simulink model "q_heli3d_skeleton_2012b"
settings: Solver=ode1  StartTime=0.0  StopTime=inf  FixedStep=0.002  RelTol=1e-3
undefined symbols (not defined in the file): A, B, C, C_0, CMD_ELEV_POS_LIMIT_LOWER, CMD_ELEV_POS_LIMIT_UPPER, CMD_RATE_LIMIT, CMD_TRAVEL_POS_LIMIT_LOWER, CMD_TRAVEL_POS_LIMIT_UPPER, elev_0, HIL, K_AMP, K_EC_E, K_EC_P, K_EC_T, K_i, K_JOYSTICK_X, K_JOYSTICK_Y, K_r, K_sf, L, qc_get_step_size, VMAX_AMP, VMAX_DAC, Vo
libraries: quarc_library x5, simulink x2, simulink_extras x2
settings Model: SimulationMode=external  ExtModeTrigDuration=500000  Creator=MLevis  LastModifiedBy=s4358046
settings SolverCC: PositivePriorityOrder=on
settings DataIOCC: LimitDataPoints=on  SaveFormat=Array  SignalLoggingSaveFormat=ModelDataLogs  ReturnWorkspaceOutputs=off
settings OptimizationCC: ExpressionDepthLimit=2147483647  InitFltsAndDblsToZero=on  LifeSpan=inf  SimCompilerOptimization=Off
settings DebuggingCC: SaveWithParameterizedLinksMsg=none  UnderspecifiedInitializationDetection=Classic  MergeDetectMultiDrivingBlocksExec=none  SolverPrmCheckMsg=warning  MultiTaskDSMMsg=warning  MultiTaskCondExecSysMsg=none  FcnCallInpInsideContextMsg=Enable All  StateNameClashWarn=warning  StrictBusMsg=None  SFUnexpectedBacktrackingDiag=warning  SFNoUnconditionalDefaultTransitionDiag=warning
settings HardwareCC: ProdBitPerPointer=32  ProdLargestAtomicFloat=None  ProdIntDivRoundTo=Undefined  ProdEndianess=Unspecified  ProdWordSize=32  ProdHWDeviceType=32-bit Generic
settings ModelReferenceCC: PropagateSignalLabelsOutOfModel=off
settings SFSimCC: SimUseLocalCustomCode=off
settings RTWCC: SystemTargetFile=quarc_win64.tlc  TemplateMakefile=quarc_default_tmf  Description=QUARC Win64 Target  ProcessScript=quarc_win64_make_rtw_hook  RTWUseLocalCustomCode=off  IncludeERTFirstTime=on  RTWCompilerOptimization=Off
settings CodeAppCC: CustomSymbolStrType=$N$R$M
settings STFCustomTargetCC: TargetPreCompLibLocation=C:\PROGRA~3\QUARC\lib\2012a\win64\release  CodeReplacementLibrary=C89/C90 (ANSI)  GeneratePreprocessorConditionals=Disable all  CombineOutputUpdateFcns=on  GRTInterface=off  SystemTargetFile=quarc_win64.tlc
settings GRTTargetCC: TargetPreCompLibLocation=C:\PROGRA~3\QUARC\lib\2012a\win64\release  CodeReplacementLibrary=C89/C90 (ANSI)  ParMdlRefBuildCompliant=off  CompOptLevelCompliant=off  ConcurrentExecutionCompliant=off  GeneratePreprocessorConditionals=Disable all  MatFileLogging=off  CPPClassGenCompliant=off  ExtMode=on  ExtModeMexFile=quarc_comm

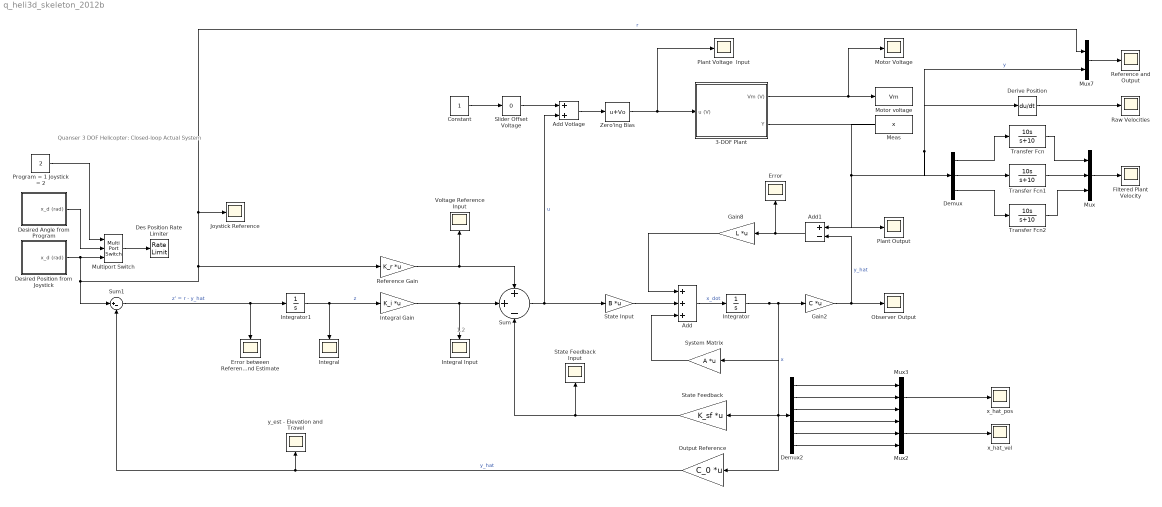
== system q_heli3d_skeleton_2012b ==
  note: Quanser 3 DOF Helicopter:
      | Closed-loop Actual System
  note: 1.2
  3-DOF Plant : Subsystem
  Add : Sum  Inputs=+++
  Add Votlage : Sum
  Add1 : Sum  Inputs=+-
  Constant : Constant
  Demux : Demux  Outputs=3
  Demux2 : Demux  Outputs=6
  Derive Position : Derivative
  Des Position Rate Limiter : RateLimiter  RisingSlewLimit=CMD_RATE_LIMIT  FallingSlewLimit=-CMD_RATE_LIMIT  SampleTimeMode=inherited
  Desired Angle from Program : Subsystem
  Desired Position from Joystick : Subsystem
  Error : Scope
      settings: TimeRange=10  YMin=-0.00225  YMax=0.002  SaveName=Error
  Error between Reference and Estimate : Scope
      settings: TimeRange=10  YMin=-0.01  YMax=0.06  SaveName=int_err
  Filtered Plant Velocity : Scope
      settings: YMin=-1.75  YMax=1.75  SaveName=y_plant_vel_filt
  Gain2 : Gain  Gain=C  Multiplication=Matrix(K*u)
  Gain8 : Gain  Gain=L  Multiplication=Matrix(K*u)
  Integral : Scope
      settings: TimeRange=10  YMin=-0.05  YMax=0.325  SaveName=int_input1
  Integral Gain : Gain  Gain=K_i  Multiplication=Matrix(K*u)
  Integral Input : Scope
      settings: TimeRange=10  YMin=-6  YMax=10  SaveName=int_input
  Integrator : Integrator
  Integrator1 : Integrator  LimitOutput=on  UpperSaturationLimit=0.7  LowerSaturationLimit=-0.7
  Joystick Reference : Scope
      settings: TimeRange=10  YMin=-0.1  YMax=2.2  SaveName=ref_info
  Meas : ToWorkspace  VariableName=x  SampleTime=-1
  Motor Voltage : Scope
      settings: YMin=-0.5  YMax=0.25  SaveName=Motor_Voltage
  Motor voltage : ToWorkspace  VariableName=Vm  SampleTime=-1
  Multiport Switch : MultiPortSwitch  Inputs=2  zeroidx=off
  Mux : Mux  Inputs=3
  Mux2 : Mux  Inputs=3
  Mux3 : Mux  Inputs=3
  Mux7 : Mux  Inputs=2
  Observer Output : Scope
      settings: TimeRange=10  YMin=-0.5  YMax=0.15  SaveName=y_est
  Output Reference : Gain  Gain=C_0  Multiplication=Matrix(K*u)
  Plant Output : Scope
      settings: YMin=-0.25  YMax=2.25  SaveName=y_plant_pos
  Plant Voltage  Input : Scope
      settings: TimeRange=10  YMin=1.3  YMax=2.9  SaveName=plnt_input
  Program = 1 Joystick = 2 : Constant  Value=2
  Raw Velocities : Scope
      settings: YMin=-0.8  YMax=0.8  SaveName=y_plant_vel
  Reference Gain : Gain  Gain=K_r  Multiplication=Matrix(K*u)
  Reference and Output : Scope
      settings: TimeRange=10  YMin=-0.1  YMax=1.2  SaveName=steady_state_error
  Slider Offset Voltage : simulink/Math Operations/Slider Gain  low=0  gain=0  high=4
  State Feedback : Gain  Gain=K_sf  Multiplication=Matrix(K*u)
  State Feedback Input : Scope
      settings: TimeRange=10  YMin=-55  YMax=55  SaveName=sf_input
  State Input : Gain  Gain=B  Multiplication=Matrix(K*u)
  Sum : Sum  Inputs=++-
  Sum1 : Sum  Inputs=|+-
  System Matrix : Gain  Gain=A  Multiplication=Matrix(K*u)
  Transfer Fcn : TransferFcn  Numerator=[10 0]  Denominator=[1 10]
  Transfer Fcn1 : TransferFcn  Numerator=[10 0]  Denominator=[1 10]
  Transfer Fcn2 : TransferFcn  Numerator=[10 0]  Denominator=[1 10]
  Voltage Reference Input : Scope
      settings: TimeRange=10  YMin=-7  YMax=-0.5  SaveName=ref_input
  Zero'ing Bias : Bias  Bias=Vo
  x_hat_pos : Scope
      settings: YMin=-0.05  YMax=0.325  SaveName=x_hat_pos
  x_hat_vel : Scope
      settings: YMin=-1.5  YMax=1.25  SaveName=x_hat_vel
  y_est - Elevation and Travel : Scope
      settings: YMin=-0.7  YMax=0.2  SaveName=y_est_e_t
  wires:
  Program = 1 Joystick = 2/1 -> Multiport Switch/1
  Desired Position from Joystick/1(x_d (rad)) -> Multiport Switch/3, Sum1/1, Mux7/1, Joystick Reference/1, Reference Gain/1  "r"
  Multiport Switch/1 -> Des Position Rate Limiter/1
  3-DOF Plant/1(Vm (V)) -> Motor voltage/1, Motor Voltage/1
  Zero'ing Bias/1 -> Plant Voltage  Input/1, 3-DOF Plant/1(u (V))
  Desired Angle from Program/1(x_d (rad)) -> Multiport Switch/2
  Transfer Fcn/1 -> Mux/1
  Demux/1 -> Transfer Fcn/1
  Demux/2 -> Transfer Fcn1/1
  Transfer Fcn1/1 -> Mux/2
  Demux/3 -> Transfer Fcn2/1
  Transfer Fcn2/1 -> Mux/3
  Mux/1 -> Filtered Plant Velocity/1
  State Input/1 -> Add/2
  Add/1 -> Integrator/1  "x_dot"
  System Matrix/1 -> Add/3
  Integrator/1 -> System Matrix/1, Gain2/1, Output Reference/1, State Feedback/1, Demux2/1  "x"
  Gain2/1 -> Observer Output/1, Add1/2  "y_hat"
  Sum/1 -> Add Votlage/2, State Input/1  "u"
  Reference Gain/1 -> Sum/1, Voltage Reference Input/1
  Add1/1 -> Gain8/1, Error/1
  Gain8/1 -> Add/1
  3-DOF Plant/2(Y) -> Meas/1, Derive Position/1, Demux/1, Mux7/2, Plant Output/1, Add1/1  "y"
  Demux2/4 -> Mux2/1
  Demux2/5 -> Mux2/2
  Demux2/6 -> Mux2/3
  Demux2/1 -> Mux3/1
  Demux2/2 -> Mux3/2
  Demux2/3 -> Mux3/3
  Mux3/1 -> x_hat_pos/1
  Mux2/1 -> x_hat_vel/1
  Derive Position/1 -> Raw Velocities/1
  Output Reference/1 -> Sum1/2, y_est - Elevation and Travel/1  "y_hat"
  Sum1/1 -> Integrator1/1, Error between Reference and Estimate/1  "z' = r - y_hat"
  State Feedback/1 -> State Feedback Input/1, Sum/3
  Integrator1/1 -> Integral/1, Integral Gain/1  "z"
  Constant/1 -> Slider Offset Voltage/1
  Add Votlage/1 -> Zero'ing Bias/1
  Slider Offset Voltage/1 -> Add Votlage/1
  Integral Gain/1 -> Integral Input/1, Sum/2
  Mux7/1 -> Reference and Output/1

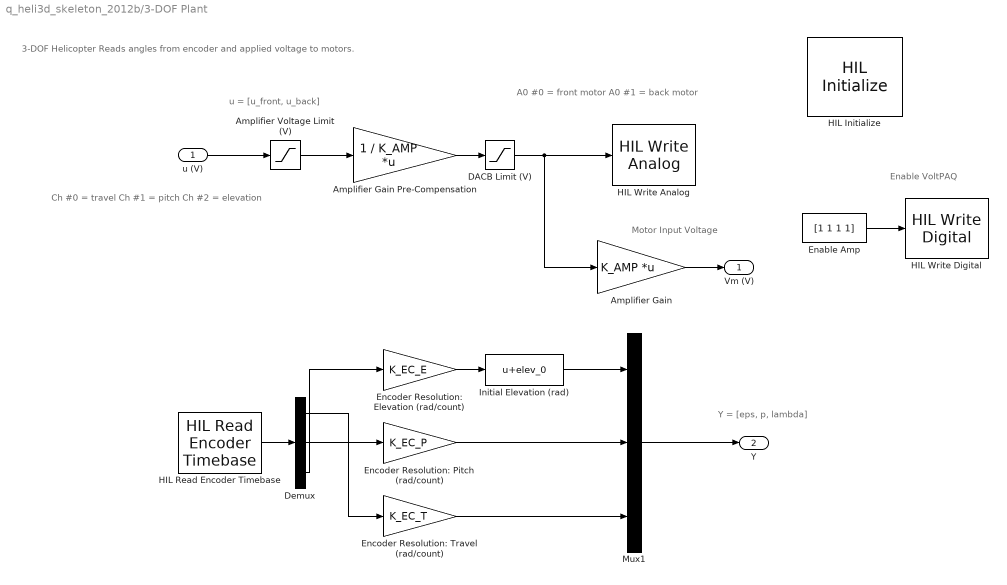
== system q_heli3d_skeleton_2012b/3-DOF Plant ==
  note: A0 #0 = front motor
      | A0 #1 = back motor
  note: u = [u_front, u_back]
  note: Motor Input Voltage
  note: 3-DOF Helicopter
      | Reads angles from encoder and applied voltage to motors.
  note: Ch #0 = travel
      | Ch #1 = pitch
      | Ch #2 = elevation
  note: Y = [eps, p, lambda]
  note: Enable VoltPAQ
  u (V) : Inport
  Amplifier Gain : Gain  Gain=K_AMP  Multiplication=Matrix(K*u)  SaturateOnIntegerOverflow=on  OutDataTypeStr=Inherit: Same as input  ParamDataTypeStr=Inherit: Same as input
  Amplifier Gain Pre-Compensation : Gain  Gain=1 / K_AMP  Multiplication=Matrix(K*u)  SaturateOnIntegerOverflow=on  OutDataTypeStr=Inherit: Same as input  ParamDataTypeStr=Inherit: Same as input
  Amplifier Voltage Limit (V) : Saturate  UpperLimit=VMAX_AMP  LowerLimit=-VMAX_AMP
  DACB Limit (V) : Saturate  UpperLimit=VMAX_DAC  LowerLimit=-VMAX_DAC
  Demux : Demux  Outputs=3
  Enable Amp : Constant  Value=[1 1 1 1]
  Encoder Resolution: Elevation (rad/count) : Gain  Gain=K_EC_E
  Encoder Resolution: Pitch (rad/count) : Gain  Gain=K_EC_P
  Encoder Resolution: Travel (rad/count) : Gain  Gain=K_EC_T
  HIL Initialize : quarc_library/Data Acquisition/Generic/Configuration/HIL Initialize  object_name=HIL-1  board_type=q8_usb  board_number=0  board_options=update_rate=normal  exclusive=off  active=on  hardware_clocks=[0:2]  clock_modes=[]  initial_clock_frequencies=[]  set_clock_params_at_start=off  set_clock_params_at_switch_in=off  set_clock_frequencies_at_start=off  set_clock_frequencies_at_switch_in=off  analog_input_channels=[0:7]  analog_input_maximums=10  analog_input_minimums=-10  set_analog_input_params_at_start=on  set_analog_input_params_at_switch_in=off  analog_output_channels=[0:7]  analog_output_maximums=10  analog_output_minimums=-10  initial_analog_outputs=[0]  final_analog_outputs=[0]  watchdog_analog_outputs=0  set_analog_output_params_at_start=on  set_analog_output_params_at_switch_in=off  set_analog_outputs_at_start=on  set_analog_outputs_at_switch_in=off  set_analog_outputs_at_terminate=on  set_analog_outputs_at_switch_out=off  set_analog_outputs_on_watchdog=off  digital_input_channels=[4:7]  digital_output_channels=[0:3]  digital_output_configuration=[]  initial_digital_outputs=[0]  final_digital_outputs=[0]  watchdog_digital_outputs=[0]  set_digital_output_params_at_start=off  set_digital_output_params_at_switch_in=off  set_digital_outputs_at_start=on  set_digital_outputs_at_switch_in=off  set_digital_outputs_at_terminate=on  set_digital_outputs_at_switch_out=off  set_digital_outputs_on_watchdog=off  encoder_channels=[0:7]  quadrature=[4]  encoder_filter_frequency=[]  initial_encoder_counts=[0]  set_encoder_params_at_start=on  set_encoder_params_at_switch_in=off  set_encoder_counts_at_start=on  set_encoder_counts_at_switch_in=off  pwm_channels=[0:7]  pwm_modes=0  pwm_frequency=99.532799999999995e6/4095  pwm_configuration=[0]  pwm_alignment=[0]  pwm_polarity=[1]  pwm_leading_deadband=[0]  pwm_trailing_deadband=[0]  initial_pwm_outputs=[0]  final_pwm_outputs=[0]  watchdog_pwm_outputs=[0]  set_pwm_params_at_start=on  set_pwm_params_at_switch_in=off  set_pwm_outputs_at_start=on  set_pwm_outputs_at_switch_in=off  set_pwm_outputs_at_terminate=on  set_pwm_outputs_at_switch_out=off  set_pwm_outputs_on_watchdog=off  other_output_channels=[]  initial_other_outputs=[]  final_other_outputs=[]  watchdog_other_outputs=[]  set_other_outputs_at_start=off  set_other_outputs_at_switch_in=off  set_other_outputs_at_terminate=off  set_other_outputs_at_switch_out=off  set_other_outputs_on_watchdog=off
  HIL Read Encoder Timebase : quarc_library/Data Acquisition/Generic/Timebases/HIL Read Encoder Timebase  object_name=HIL-1  clock=0  channels=[0,1,2]  samples_in_buffer=max(ceil(1/qc_get_step_size), 1)  active=on  vector_output=on  data_type_mode=Inherit via back propagation  data_type=double
  HIL Write Analog : quarc_library/Data Acquisition/Generic/Immediate I//O/HIL Write Analog  object_name=HIL-1  channels=[0,1]  sample_time=-1  active=off  vector_input=on
  HIL Write Digital : quarc_library/Data Acquisition/Generic/Immediate I//O/HIL Write Digital  object_name=HIL-1  channels=[0:3]  sample_time=-1  active=off  vector_input=on
  Initial Elevation (rad) : Bias  Bias=elev_0
  Mux1 : Mux  Inputs=3
  Vm (V) : Outport
  Y : Outport  Port=2
  wires:
  HIL Read Encoder Timebase/1 -> Demux/1
  Mux1/1 -> Y/1
  Amplifier Gain Pre-Compensation/1 -> DACB Limit (V)/1
  Amplifier Voltage Limit (V)/1 -> Amplifier Gain Pre-Compensation/1
  Amplifier Gain/1 -> Vm (V)/1
  u (V)/1 -> Amplifier Voltage Limit (V)/1
  DACB Limit (V)/1 -> Amplifier Gain/1, HIL Write Analog/1
  Demux/3 -> Encoder Resolution: Elevation (rad/count)/1
  Demux/1 -> Encoder Resolution: Travel (rad/count)/1
  Demux/2 -> Encoder Resolution: Pitch (rad/count)/1
  Encoder Resolution: Elevation (rad/count)/1 -> Initial Elevation (rad)/1
  Encoder Resolution: Pitch (rad/count)/1 -> Mux1/2
  Encoder Resolution: Travel (rad/count)/1 -> Mux1/3
  Initial Elevation (rad)/1 -> Mux1/1
  Enable Amp/1 -> HIL Write Digital/1

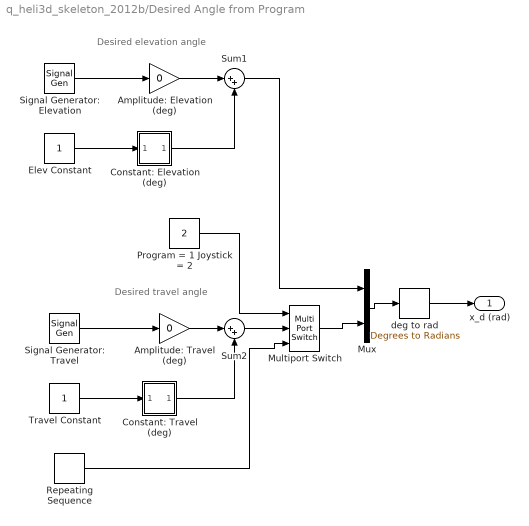
== system q_heli3d_skeleton_2012b/Desired Angle from Program ==
  note: Desired travel angle
  note: Desired elevation angle
  Amplitude: Elevation (deg) : Gain  Gain=0
  Amplitude: Travel (deg) : Gain  Gain=0
  Constant: Elevation (deg) : Subsystem  LoadFcn=slideg Load  StartFcn=slideg StartFcn  StopFcn=slideg StopFcn  mask(Slider Gain){low=-27.5, gain=-27.5, high=30}
      settings: CopyFcn=slideg Copy  DeleteFcn=slideg DeleteBlock  NameChangeFcn=slideg NameChange  OpenFcn=slideg Open  CloseFcn=slideg Close  ParentCloseFcn=slideg ParentClose
      mask Display: disp(gain)
  Constant: Travel (deg) : Subsystem  LoadFcn=slideg Load  StartFcn=slideg StartFcn  StopFcn=slideg StopFcn  mask(Slider Gain){low=-90, gain=0, high=90}
      settings: CopyFcn=slideg Copy  DeleteFcn=slideg DeleteBlock  NameChangeFcn=slideg NameChange  OpenFcn=slideg Open  CloseFcn=slideg Close  ParentCloseFcn=slideg ParentClose
      mask Display: disp(gain)
  Elev Constant : Constant
  Multiport Switch : MultiPortSwitch  Inputs=2  zeroidx=off
  Mux : Mux  Inputs=2
  Program = 1 Joystick = 2 : Constant  Value=2
  Repeating Sequence : simulink/Sources/Repeating Sequence  rep_seq_t="[0  15 16  30  45  46 60 ]"  rep_seq_y="[0 0 30 30  30 0 0 ]"
  Signal Generator: Elevation : SignalGenerator  WaveForm=square  Frequency=0.04
  Signal Generator: Travel : SignalGenerator  WaveForm=square  Frequency=0.03
  Sum1 : Sum  Inputs=|++
  Sum2 : Sum  Inputs=|++
  Travel Constant : Constant
  deg to rad : simulink_extras/Transformations/Degrees to Radians
  x_d (rad) : Outport
  wires:
  deg to rad/1 -> x_d (rad)/1
  Signal Generator: Travel/1 -> Amplitude: Travel (deg)/1
  Amplitude: Travel (deg)/1 -> Sum2/1
  Travel Constant/1 -> Constant: Travel (deg)/1(In1)
  Sum1/1 -> Mux/1
  Signal Generator: Elevation/1 -> Amplitude: Elevation (deg)/1
  Amplitude: Elevation (deg)/1 -> Sum1/1
  Mux/1 -> deg to rad/1
  Elev Constant/1 -> Constant: Elevation (deg)/1(In1)
  Constant: Elevation (deg)/1(Out1) -> Sum1/2
  Constant: Travel (deg)/1(Out1) -> Sum2/2
  Sum2/1 -> Multiport Switch/2
  Repeating Sequence/1 -> Multiport Switch/3
  Multiport Switch/1 -> Mux/2
  Program = 1 Joystick = 2/1 -> Multiport Switch/1

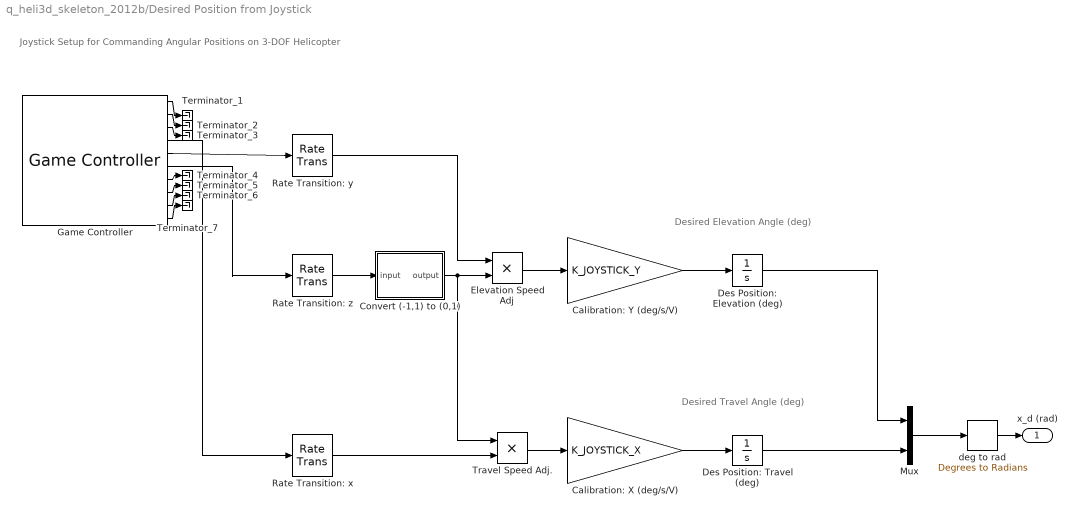
== system q_heli3d_skeleton_2012b/Desired Position from Joystick ==
  note: Desired Elevation Angle (deg)
  note: Desired Travel Angle (deg)
  note: Joystick Setup for Commanding Angular Positions on 3-DOF Helicopter
  Calibration: X (deg/s/V) : Gain  Gain=K_JOYSTICK_X
  Calibration: Y (deg/s/V) : Gain  Gain=K_JOYSTICK_Y
  Convert (-1,1) to (0,1) : Subsystem
  Des Position: Elevation (deg) : Integrator  InitialCondition=elev_0*180/pi  LimitOutput=on  UpperSaturationLimit=CMD_ELEV_POS_LIMIT_UPPER  LowerSaturationLimit=CMD_ELEV_POS_LIMIT_LOWER
  Des Position: Travel (deg) : Integrator  UpperSaturationLimit=CMD_TRAVEL_POS_LIMIT_UPPER  LowerSaturationLimit=CMD_TRAVEL_POS_LIMIT_LOWER
  Elevation Speed Adj : Product  RndMeth=Zero
  Game Controller : quarc_library/Devices/Peripherals/Target/Game Controller  controller=1  buffer_size=12  deadzone=[]  saturation=[]  sample_time=max(qc_get_step_size, 0.01)  auto_center=off  enabled=on
  Mux : Mux  Inputs=2
  Rate Transition: x : RateTransition
  Rate Transition: y : RateTransition
  Rate Transition: z : RateTransition
  Terminator_{1..7} (7 alike) : Terminator
  Travel Speed Adj. : Product  RndMeth=Zero
  deg to rad : simulink_extras/Transformations/Degrees to Radians
  x_d (rad) : Outport
  wires:
  Des Position: Elevation (deg)/1 -> Mux/1
  Mux/1 -> deg to rad/1
  deg to rad/1 -> x_d (rad)/1
  Calibration: X (deg/s/V)/1 -> Des Position: Travel (deg)/1
  Travel Speed Adj./1 -> Calibration: X (deg/s/V)/1
  Elevation Speed Adj/1 -> Calibration: Y (deg/s/V)/1
  Calibration: Y (deg/s/V)/1 -> Des Position: Elevation (deg)/1
  Convert (-1,1) to (0,1)/1(output) -> Travel Speed Adj./1, Elevation Speed Adj/2
  Rate Transition: z/1 -> Convert (-1,1) to (0,1)/1(input)
  Rate Transition: y/1 -> Elevation Speed Adj/1
  Rate Transition: x/1 -> Travel Speed Adj./2
  Game Controller/5 -> Rate Transition: y/1
  Game Controller/6 -> Rate Transition: z/1
  Game Controller/4 -> Rate Transition: x/1
  Game Controller/1 -> Terminator_1/1
  Game Controller/2 -> Terminator_2/1
  Game Controller/3 -> Terminator_3/1
  Game Controller/7 -> Terminator_4/1
  Game Controller/8 -> Terminator_5/1
  Game Controller/9 -> Terminator_6/1
  Game Controller/10 -> Terminator_7/1
  Des Position: Travel (deg)/1 -> Mux/2

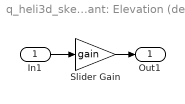
== system q_heli3d_skeleton_2012b/Desired Angle from Program/Constant: Elevation (deg) ==
  In1 : Inport
  Slider Gain : Gain  Gain=gain  SaturateOnIntegerOverflow=on  OutDataTypeStr=Inherit: Same as input  ParamDataTypeStr=Inherit: Same as input
  Out1 : Outport
  wires:
  In1/1 -> Slider Gain/1
  Slider Gain/1 -> Out1/1

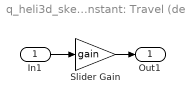
== system q_heli3d_skeleton_2012b/Desired Angle from Program/Constant: Travel (deg) ==
  In1 : Inport
  Slider Gain : Gain  Gain=gain  SaturateOnIntegerOverflow=on  OutDataTypeStr=Inherit: Same as input  ParamDataTypeStr=Inherit: Same as input
  Out1 : Outport
  wires:
  In1/1 -> Slider Gain/1
  Slider Gain/1 -> Out1/1

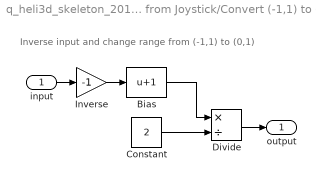
== system q_heli3d_skeleton_2012b/Desired Position from Joystick/Convert (-1,1) to (0,1) ==
  note: Inverse input and change range from (-1,1) to (0,1)
  input : Inport
  Bias : Bias  Bias=1
  Constant : Constant  Value=2
  Divide : Product  Inputs=*/
  Inverse : Gain  Gain=-1
  output : Outport
  wires:
  Constant/1 -> Divide/2
  Bias/1 -> Divide/1
  input/1 -> Inverse/1
  Divide/1 -> output/1
  Inverse/1 -> Bias/1
